simulink model "untitled1"  (R2023b)
settings: Solver=VariableStepAuto  StartTime=0.0  StopTime=1000  RelTol=1e-3
values from neighbouring files (symbols this model uses):
  Hp = Kp /( Tp *s  +1)    [test.m]
  Hr = Hd/ Hf    [test.m]
settings Model: Creator=wombelbat  LastModifiedBy=wombelbat

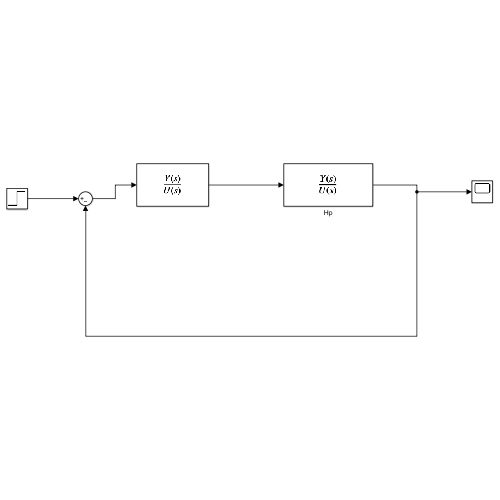
[thumbnail: Simulink's stored preview of the top-level diagram]
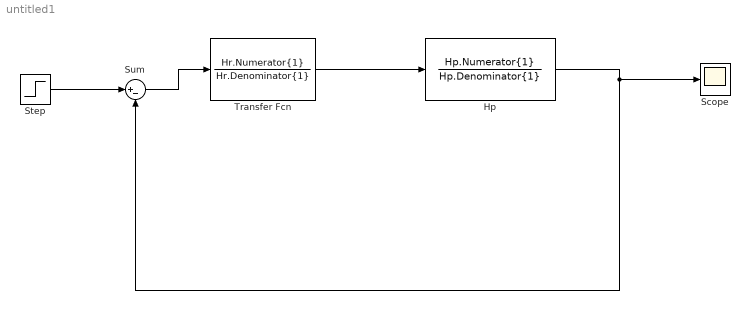
== system untitled1 ==
  Hp : TransferFcn  Numerator=Hp.Numerator{1}  Denominator=Hp.Denominator{1}
  Scope : Scope
  Step : Step  After=87  SampleTime=0
  Sum : Sum  Inputs=|+-
  Transfer Fcn : TransferFcn  Numerator=Hr.Numerator{1}  Denominator=Hr.Denominator{1}
  wires:
  Hp/1 -> Sum/2, Scope/1
  Step/1 -> Sum/1
  Sum/1 -> Transfer Fcn/1
  Transfer Fcn/1 -> Hp/1
